simulink model "ergasia1"  (R2019a)
settings: Solver=VariableStepAuto  StartTime=0.0  StopTime=1  RelTol=1e-3
libraries: dspstat3 x1
settings Model: Creator=giannis  LastModifiedBy=giannis

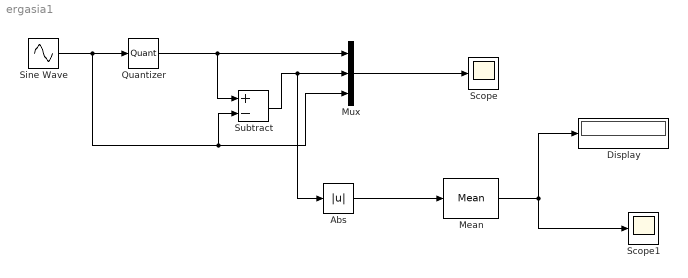
== system ergasia1 ==
  Abs : Abs
  Display : Display
  Mean : dspstat3/Mean  run=on  InputProcessing=Columns as channels (frame based)  reset_popup=None  directionMode=Each column  dimension=1  roiEnable=off  roiType=Rectangles  roiPortion=Entire ROI  roiOutput=Individual statistics for each ROI  roiFlag=off  roundingMode=Floor  overflowMode=off  outputDataTypeStr=Inherit: Same as accumulator  outputMin=[]  outputMax=[]  outputLastDataTypeStr=Inherit: Same as accumulator
  Mux : Mux  Inputs=3
  Quantizer : Quantizer  QuantizationInterval=16/(2^2)  SampleTime=1/(2.5*10^3)
  Scope : Scope
  Scope1 : Scope
  Sine Wave : Sin  Amplitude=8  Frequency=2*pi*2000  Phase=1  SampleTime=1*10^(-6)
  Subtract : Sum  Inputs=+-
  wires:
  Sine Wave/1 -> Subtract/2, Mux/3, Quantizer/1
  Quantizer/1 -> Subtract/1, Mux/1
  Subtract/1 -> Abs/1, Mux/2
  Mux/1 -> Scope/1
  Abs/1 -> Mean/1
  Mean/1 -> Display/1, Scope1/1
